simulink model "example_2_attitude"  (R2016a)
settings: Solver=VariableStepAuto  StartTime=0.0  StopTime=Tsim  RelTol=1e-3
values from neighbouring files (symbols this model uses):
  qr = qr./norm(qr)    [init_A.m]    (also in init_B.m)
  ref_A = [pi, pi, pi]    [init_A.m]    (also in init_B.m)
  ref_b = [0, 0, 0]    [init_A.m]    (also in init_B.m)
  ref_p = [1, 2, 3]    [init_A.m]    (also in init_B.m)
  ref_w = [1, 1.5, 2]    [init_A.m]    (also in init_B.m)
  sequence = 1    [init_A.m]    (also in init_B.m = 2)
libraries: aerolibtransform2 x4, aerolibutil x1
settings Model: Creator=mgreiff  LastModifiedBy=mgreiff

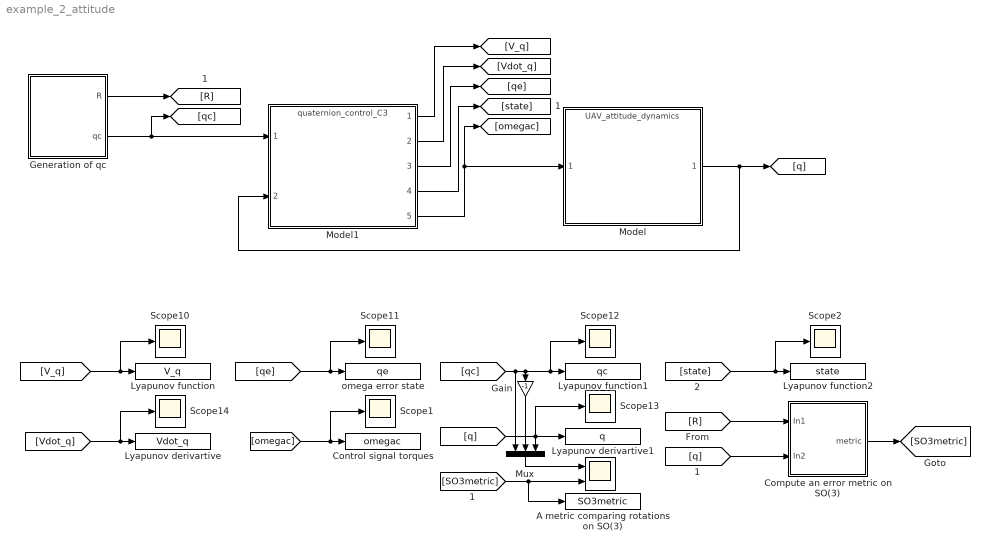
== system example_2_attitude ==
  "                                     " : Scope  NumInputPorts=2
  A metric comparing rotations on SO(3) : ToWorkspace  VariableName=SO3metric  SaveFormat=Timeseries  SampleTime=-1
  Compute an error metric on SO(3) : Subsystem
  Control signal torques : ToWorkspace  VariableName=omegac  SaveFormat=Timeseries  SampleTime=-1
  Gain : Gain  Gain=-1
  Generation of qc : Subsystem
  Lyapunov derivartive : ToWorkspace  VariableName=Vdot_q  SaveFormat=Timeseries  SampleTime=-1
  Lyapunov derivartive1 : ToWorkspace  VariableName=q  SaveFormat=Timeseries  SampleTime=-1
  Lyapunov function : ToWorkspace  VariableName=V_q  SaveFormat=Timeseries  SampleTime=-1
  Lyapunov function1 : ToWorkspace  VariableName=qc  SaveFormat=Timeseries  SampleTime=-1
  Lyapunov function2 : ToWorkspace  VariableName=state  SaveFormat=Timeseries  SampleTime=-1
  Model : ModelReference  ModelNameDialog=UAV_attitude_dynamics.slx  SimulationMode=Normal  ModelReferenceVersion=1.15
  Model1 : ModelReference  ModelNameDialog=quaternion_control_C3.slx  SimulationMode=Normal  ModelReferenceVersion=1.25
  Mux : Mux  Inputs=3
  Scope{1..2,10..14} (7 alike) : Scope
  omega error state : ToWorkspace  VariableName=qe  SaveFormat=Timeseries  SampleTime=-1
  wires:
  Generation of qc/2("qc ") -> [qc], Model1/1
  [V_q] -> Lyapunov function/1, Scope10/1
  [Vdot_q] -> Lyapunov derivartive/1, Scope14/1
  [qc] -> Gain/1, Lyapunov function1/1, Scope12/1, Mux/1
  [q] -> Mux/3, Lyapunov derivartive1/1, Scope13/1
  [qe] -> omega error state/1, Scope11/1
  Model1/1 -> [V_q]
  Model1/2 -> [Vdot_q]
  Model1/3 -> [qe]
  Mux/1 -> "                                     "/1
  [omegac] -> Control signal torques/1, Scope1/1
  Generation of qc/1(R) -> [R]
  [R] -> Compute an error metric on SO(3)/1(In1)
  [q] -> Compute an error metric on SO(3)/2(In2)
  Compute an error metric on SO(3)/1(metric) -> [SO3metric]
  [SO3metric] -> A metric comparing rotations on SO(3)/1, "                                     "/2
  Model1/5 -> [omegac], Model/1
  [state] -> Lyapunov function2/1, Scope2/1
  Model1/4 -> [state]
  Model/1 -> Model1/2, [q]
  Gain/1 -> Mux/2

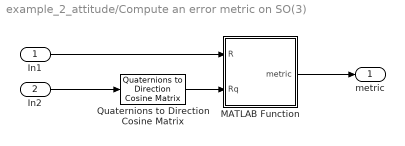
== system example_2_attitude/Compute an error metric on SO(3) ==
  In1 : Inport
  In2 : Inport  Port=2
  MATLAB Function : MATLAB Function  TreatAsAtomicUnit=on
  Quaternions to Direction Cosine Matrix : aerolibtransform2/Quaternions to  Direction Cosine Matrix
  metric : Outport
  wires:
  MATLAB Function/1(metric) -> metric/1
  Quaternions to Direction Cosine Matrix/1 -> MATLAB Function/2(Rq)
  In1/1 -> MATLAB Function/1(R)
  In2/1 -> Quaternions to Direction Cosine Matrix/1

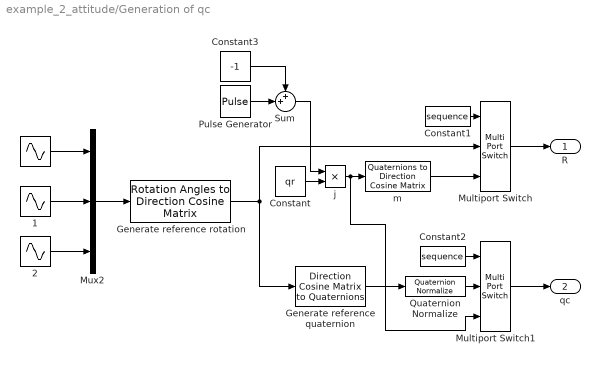
== system example_2_attitude/Generation of qc ==
  " " : Sin  Amplitude=ref_A(1)  Bias=ref_b(1)  Frequency=ref_w(1)  Phase=ref_p(1)  SampleTime=0.001
  " 1" : Sin  Amplitude=ref_A(2)  Bias=ref_b(2)  Frequency=ref_w(2)  Phase=ref_p(2)  SampleTime=0.001
  " 2" : Sin  Amplitude=ref_A(3)  Bias=ref_b(3)  Frequency=ref_w(3)  Phase=ref_p(3)  SampleTime=0.001
  Constant : Constant  Value=qr
  Constant1 : Constant  Value=sequence
  Constant2 : Constant  Value=sequence
  Constant3 : Constant  Value=-1
  Generate reference quaternion : aerolibtransform2/Direction Cosine Matrix  to Quaternions
  Generate reference rotation : aerolibtransform2/Rotation Angles to Direction Cosine Matrix  rotationOrder=ZYX
  Multiport Switch : MultiPortSwitch  Inputs=2
  Multiport Switch1 : MultiPortSwitch  Inputs=2
  Mux2 : Mux  Inputs=3
  Pulse Generator : DiscretePulseGenerator  PulseType=Time based  Amplitude=2  Period=1  PulseWidth=50
  Quaternion Normalize : aerolibutil/Quaternion Normalize
  Sum : Sum  Inputs=++|
  j : Product
  m : aerolibtransform2/Quaternions to  Direction Cosine Matrix
  R : Outport
  "qc " : Outport  Port=2
  wires:
  " 1"/1 -> Mux2/2
  " "/1 -> Mux2/1
  " 2"/1 -> Mux2/3
  Generate reference rotation/1 -> Multiport Switch/2, Generate reference quaternion/1
  Mux2/1 -> Generate reference rotation/1
  Multiport Switch/1 -> R/1
  m/1 -> Multiport Switch/3
  Multiport Switch1/1 -> "qc "/1
  Generate reference quaternion/1 -> Quaternion Normalize/1
  Constant1/1 -> Multiport Switch/1
  Constant2/1 -> Multiport Switch1/1
  Quaternion Normalize/1 -> Multiport Switch1/2
  Pulse Generator/1 -> Sum/2
  Constant3/1 -> Sum/1
  Sum/1 -> j/1
  Constant/1 -> j/2
  j/1 -> Multiport Switch1/3, m/1

== matlab function example_2_attitude/Compute an error metric on SO(3)/MATLAB Function ==
  data: R input; metric output; Rq input
function metric = fcn(R, Rq)
%#codegen
metric = trace(eye(3) - Rq'*R);
end
